simulink model "parte1_eje13_controlPI"  (R2017b)
settings: Solver=VariableStepAuto  StartTime=0.0  StopTime=20  RelTol=1e-3
libraries: simulink x1
settings Model: Creator=cjuar  LastModifiedBy=cjuar

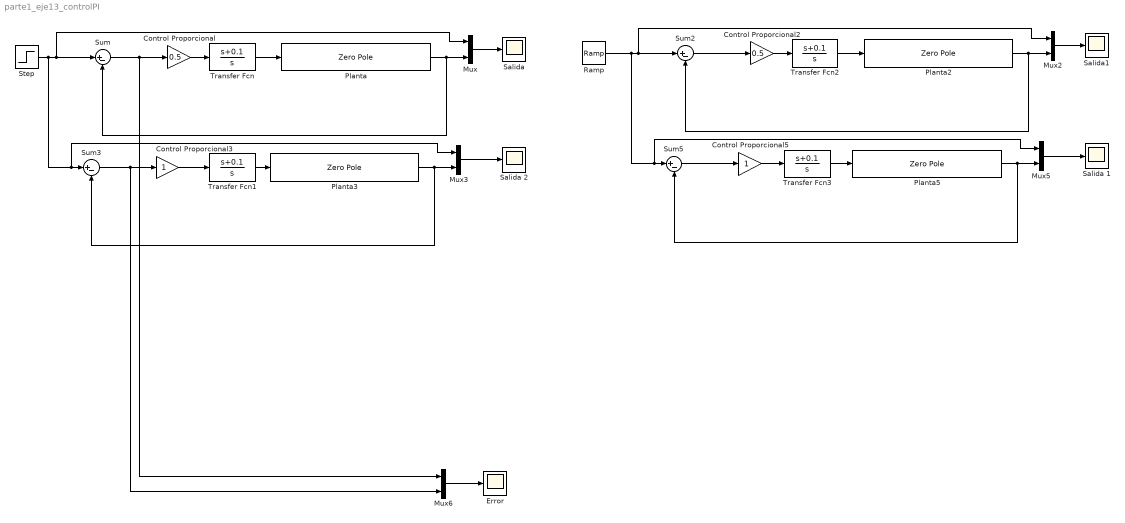
== system parte1_eje13_controlPI ==
  Control Proporcional : Gain  Gain=0.5
  Control Proporcional2 : Gain  Gain=0.5
  Control Proporcional3 : Gain
  Control Proporcional5 : Gain
  Error : Scope
  Mux{,2..3,5..6} (5 alike) : Mux  Inputs=2
  Planta{,2..3,5} (4 alike) : ZeroPole  Zeros=[]  Poles=[0 -6 -18]  Gain=1080
  Ramp : simulink/Sources/Ramp  slope=1  start=0  X0=0
  Salida : Scope
  Salida 1 : Scope
  Salida 2 : Scope
  Salida1 : Scope
  Step : Step  SampleTime=0
  Sum{,2..3,5} (4 alike) : Sum  Inputs=|+-
  Transfer Fcn{,1..3} (4 alike) : TransferFcn  Numerator=[1 0.1]  Denominator=[1 0]
  wires:
  Control Proporcional/1 -> Transfer Fcn/1
  Sum/1 -> Control Proporcional/1, Mux6/1
  Planta/1 -> Sum/2, Mux/2
  Mux/1 -> Salida/1
  Step/1 -> Mux3/1, Sum3/1, Mux/1, Sum/1
  Mux3/1 -> Salida 2/1
  Planta3/1 -> Mux3/2, Sum3/2
  Sum3/1 -> Mux6/2, Control Proporcional3/1
  Control Proporcional3/1 -> Transfer Fcn1/1
  Sum2/1 -> Control Proporcional2/1
  Control Proporcional2/1 -> Transfer Fcn2/1
  Planta2/1 -> Sum2/2, Mux2/2
  Ramp/1 -> Mux5/1, Sum5/1, Mux2/1, Sum2/1
  Sum5/1 -> Control Proporcional5/1
  Control Proporcional5/1 -> Transfer Fcn3/1
  Planta5/1 -> Mux5/2, Sum5/2
  Mux5/1 -> Salida 1/1
  Mux2/1 -> Salida1/1
  Mux6/1 -> Error/1
  Transfer Fcn/1 -> Planta/1
  Transfer Fcn1/1 -> Planta3/1
  Transfer Fcn2/1 -> Planta2/1
  Transfer Fcn3/1 -> Planta5/1
